simulink model "AppLogicDesign"  (R2019a)
settings: Solver=VariableStepAuto  StartTime=0.0  StopTime=10.0  RelTol=1e-3
settings Model: Creator=G5  LastModifiedBy=G5

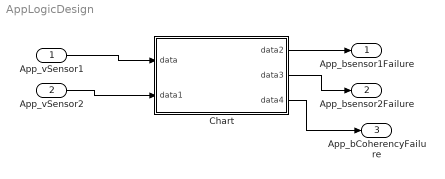
== system AppLogicDesign ==
  App_vSensor1 : Inport
  App_vSensor2 : Inport  Port=2
  Chart : Stateflow chart  BlockKeywords=__PRM__SERIALIZED__DATA__:Stateflow Chart,Stateflow Diagram  TreatAsAtomicUnit=on
  App_bsensor1Failure : Outport
  App_bsensor2Failure : Outport  Port=2
  App_bCoherencyFailure : Outport  Port=3
  wires:
  App_vSensor1/1 -> Chart/1(data)
  App_vSensor2/1 -> Chart/2(data1)
  Chart/1(data2) -> App_bsensor1Failure/1
  Chart/2(data3) -> App_bsensor2Failure/1
  Chart/3(data4) -> App_bCoherencyFailure/1

== stateflow chart AppLogicDesign/Chart ==
  (default) -> (junction 45) : % SenCheck
  (junction 45) -> (junction 46) [order 1] : [App_vSensor1 >= 0.5 && App_vSensor1 <= 4.5]
  (junction 45) -> (junction 47) [order 2] : {App_bsensor1Failure = 1;}
  (junction 46) -> (junction 48) : {App_bsensor1Failure = 0;}
  (junction 48) -> (junction 47)
  (junction 47) -> (junction 56)
  (junction 56) -> (junction 57) [order 1] : [App_vSensor2 >= 0.5 && App_vSensor2 <= 4.5]
  (junction 56) -> (junction 58) [order 2] : {App_bsensor2Failure = 1;}
  (junction 57) -> (junction 59) : {App_bsensor2Failure = 0;}
  (junction 59) -> (junction 58)
  (junction 58) -> (junction 67)
  (junction 67) -> (junction 68) [order 1] : [App_vSensor1 + App_vSensor2 == 5]
  (junction 67) -> (junction 69) [order 2] : {App_bCoherencyFailure = 1;}
  (junction 68) -> (junction 70) : {App_bCoherencyFailure = 0;}
  (junction 70) -> (junction 69)
  (junction 69) -> (junction 71)
  data: data input; data1 input; data2 output; data3 output; data4 output
